simulink model "Demo1"  (R2015a)
settings: Solver=ode45  StartTime=0.0  StopTime=10.0  RelTol=1e-3
InitFcn:
  | Initilization_simulink
values from neighbouring files (symbols this model uses):
  ref = [4.07104996922  -4.5013493727  0; -4.9106735029  -4.17473684081  0; 5.68808751891  0.810273345356  0]    [Config.mat]
undefined symbols (not defined in the file or in its folder): IsPositionTracked, IsSkeletonTracked, JointDepthIndices, JointImageIndices, JointTrackingState, JointWorldCoordinates, none, PositionDepthIndices, PositionImageIndices, PositionWorldCoordinates, SegmentationData, SkeletonTrackingID, videoinput
libraries: imaqlib x1, visionsinks x1
settings Model: CovSFcnEnable=off  Creator=tzwijger  LastModifiedBy=tzwijger
settings DebuggingCC: SolverPrmCheckMsg=warning

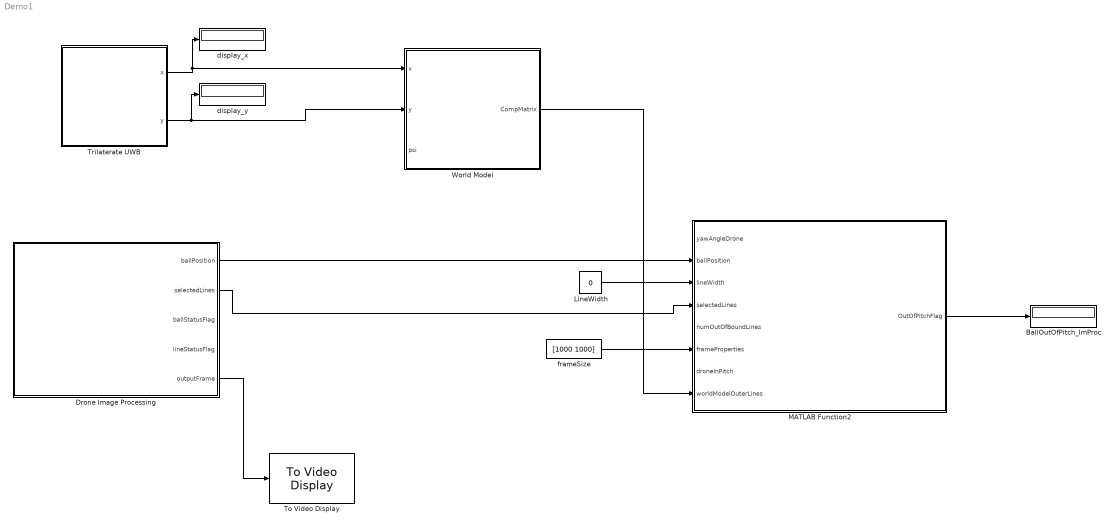
== system Demo1 ==
  BallOutOfPitch_ImProc : Display
  Drone Image Processing : Subsystem
  LineWidth : Constant  Value=0
  MATLAB Function2 : MATLAB Function  TreatAsAtomicUnit=on
  To Video Display : visionsinks/To Video Display  windowSizeMode=True size (1:1)  openAtMdlStart=on  fullScreen=off  videoWindowX=40  videoWindowY=53  saveWindowSize=off  videoWindowWidth=132  videoWindowHeight=41  inputColorFormat=RGB  inputType=Obsolete  imagePorts=One multidimensional signal  OutputDevice=On-screen video monitor  dataOrg=Column-major  isWindowOpen=off
  Trilaterate UWB : Subsystem
  World Model : Subsystem
  display_x : Display
  display_y : Display
  frameSize : Constant  Value=[1000 1000]
  wires:
  Trilaterate UWB/1(x) -> display_x/1, World Model/1(x)
  Trilaterate UWB/2(y) -> World Model/2(y), display_y/1
  Drone Image Processing/5(outputFrame) -> To Video Display/1
  Drone Image Processing/1("ballPosition ") -> MATLAB Function2/2(ballPosition)
  ? -> World Model/3(psi), MATLAB Function2/1(yawAngleDrone)
  LineWidth/1 -> MATLAB Function2/3(lineWidth)
  frameSize/1 -> MATLAB Function2/6(frameProperties)
  ? -> MATLAB Function2/7(droneInPitch)
  MATLAB Function2/1(OutOfPitchFlag) -> BallOutOfPitch_ImProc/1
  Drone Image Processing/2(selectedLines) -> MATLAB Function2/4(selectedLines)
  World Model/1(CompMatrix) -> MATLAB Function2/8(worldModelOuterLines)

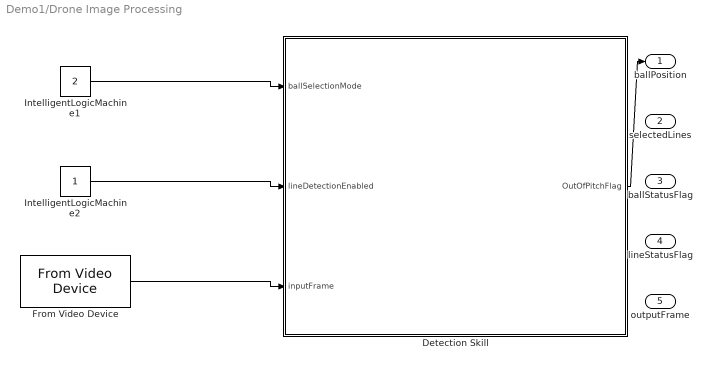
== system Demo1/Drone Image Processing ==
  Detection Skill : MATLAB Function  TreatAsAtomicUnit=on
  From Video Device : imaqlib/From Video Device  DeviceMenu=(none)  Device=winvideo 1 (HP HD Webcam)  ObjConstructor=videoinput('winvideo', 1)  VideoFormatMenu=(none)  VideoFormat=RGB24_640x480  VideoSource=input1  ROIPosition=[0 0 480 640]  EnableHWTrigger=off  TriggerConfiguration=none/none  SampleTime=1/30  OutputPortsMode=One multidimensional signal  DataType=single  CanDoHWTrigger=no  ReturnedColorSpace=rgb  BlockHandle=1921.0006  ROIWidth=640  ROIHeight=480  ROIColumn=0  ROIRow=0  EngXMLPath=C:\Program Files\MATLAB\R2015a\toolbox\imaq\imaq\private  DevXMLPath=C:\Program Files\MATLAB\R2015a\toolbox\imaq\imaqadaptors\win64  EngLibPath=C:\Program Files\MATLAB\R2015a\toolbox\imaq\imaqblks\imaqmex\win64  ColorSpace=rgb  BayerSensorAlignment=grbg  AllMetadata=IsPositionTracked;IsSkeletonTracked;JointDepthIndices;JointImageIndices;JointTrackingState;JointWorldCoordinates;PositionDepthIndices;PositionImageIndices;PositionWorldCoordinates;SegmentationData;SkeletonTrackingID
  IntelligentLogicMachine1 : Constant  Value=2
  IntelligentLogicMachine2 : Constant
  "ballPosition " : Outport
  selectedLines : Outport  Port=2
  ballStatusFlag : Outport  Port=3
  lineStatusFlag : Outport  Port=4
  outputFrame : Outport  Port=5
  wires:
  Detection Skill/1(OutOfPitchFlag) -> "ballPosition "/1
  ? -> outputFrame/1
  ? -> ballStatusFlag/1
  ? -> lineStatusFlag/1
  ? -> selectedLines/1
  IntelligentLogicMachine1/1 -> Detection Skill/1(ballSelectionMode)
  From Video Device/1 -> Detection Skill/3(inputFrame)
  IntelligentLogicMachine2/1 -> Detection Skill/2(lineDetectionEnabled)

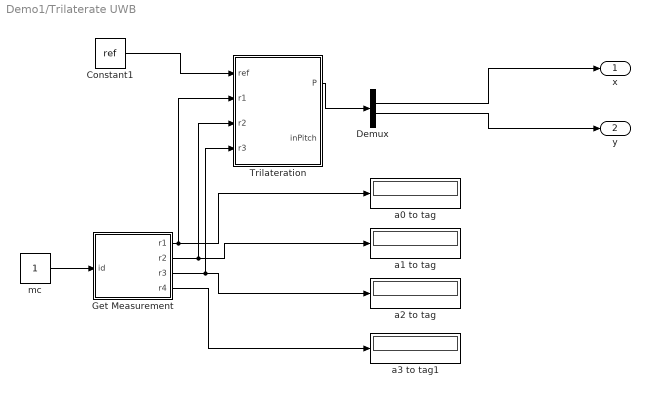
== system Demo1/Trilaterate UWB ==
  Constant1 : Constant  Value=ref
  Demux : Demux
  Get Measurement : MATLAB Function  TreatAsAtomicUnit=on
  Trilateration : MATLAB Function  TreatAsAtomicUnit=on
  a0 to tag : Display
  a1 to tag : Display
  a2 to tag : Display
  a3 to tag1 : Display
  mc : Constant
  x : Outport
  y : Outport  Port=2
  wires:
  Demux/3 -> y/1
  Demux/2 -> x/1
  Trilateration/1(P) -> Demux/1
  Constant1/1 -> Trilateration/1(ref)
  Get Measurement/3(r3) -> a2 to tag/1, Trilateration/4(r3)
  Get Measurement/2(r2) -> a1 to tag/1, Trilateration/3(r2)
  mc/1 -> Get Measurement/1(id)
  Get Measurement/1(r1) -> Trilateration/2(r1), a0 to tag/1
  Get Measurement/4(r4) -> a3 to tag1/1

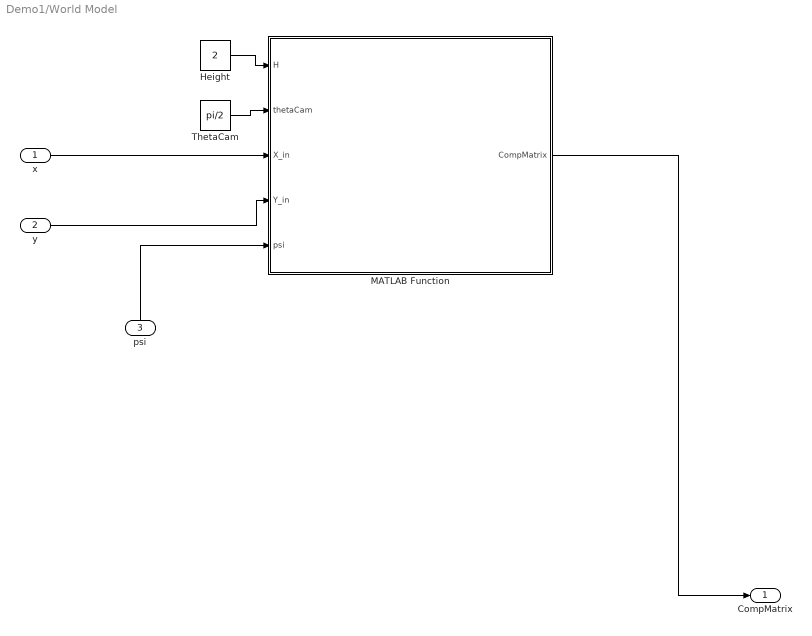
== system Demo1/World Model ==
  x : Inport
  y : Inport  Port=2
  psi : Inport  Port=3
  Height : Constant  Value=2
  MATLAB Function : MATLAB Function  TreatAsAtomicUnit=on
  ThetaCam : Constant  Value=pi/2
  CompMatrix : Outport
  wires:
  MATLAB Function/1(CompMatrix) -> CompMatrix/1
  ThetaCam/1 -> MATLAB Function/2(thetaCam)
  x/1 -> MATLAB Function/3(X_in)
  y/1 -> MATLAB Function/4(Y_in)
  psi/1 -> MATLAB Function/5(psi)
  Height/1 -> MATLAB Function/1(H)

== matlab function Demo1/Trilaterate UWB/Trilateration ==
  data: P output; ref input; r1 input; r2 input; r3 input; inPitch output
function [P, inPitch] = trilateration(ref,r1,r2,r3)%,fign,field2im_params)
% persistent plots k nrplots

coder.extrinsic('Trilateration')

% if isempty(plots)
%     plots = [0];
%     k = 1;
%     nrplots = 10;
% end

P = zeros(4,1);
P = Trilateration(ref',[r1 r2 r3],eye(3));

% % Plot and print results
% [plots, k] = update_plot_trilat(plots, k, fign, P(2:3), field2im_params, nrplots);

== matlab function Demo1/Trilaterate UWB/Get Measurement ==
  data: id input; r1 output; r2 output; r3 output; r4 output
function [r1,r2,r3,r4] = GetMC_sm(id) 
    % Input: Serial Port to A0
    %        
    % Output: Raw data for triangulation
    %
    % Message syntax is explained in the Decawave documentation
    % DecaRangeRTLS_PC_Source_Code_Guide.pdf  - Section 2.3.2
    % DecaRangeRTLS_ARM_Source_Code_Guide.pdf - Section 2.6

    % Make sure to get a measurement with the correct identifier
    persistent s;
    %coder.extrinsic('instrfind','delete','serial','fscanf','strsplit')
    coder.extrinsic('instrfind','delete','serial','fscanf','GetMC')
    
    r1 = 0; r2 = 0; r3 = 0; r4 = 0;
    
    if isempty(s)
        ports = instrfind;
        if ~isempty(ports)
            fclose(ports);
            delete(ports);
        end
        % Establish new connection
        s = serial('COM33','BaudRate',9600,'Parity','None');

        % Open connection
        fopen(s);
        fscanf(s); % Get init mc out of the way and test connection
    end
    
    ids = ['mc';'mr';'ma'];
    id = ids(id,:);
    
    dist = zeros(1,4);
    dist = GetMC(s,id);
    r1 = dist(1);
    r2 = dist(2);
    r3 = dist(3);
    r4 = dist(4); 
end

== matlab function Demo1/World Model/MATLAB Function ==
  data: H input; CompMatrix output; thetaCam input; X_in input; Y_in input; psi input
function CompMatrix   = World(H,thetaCam,X_in,Y_in,psi)

% %field line numbering:  222222222222222222223
%                         1                   3
%                         1                   3
%                         1                   3
%                         1                   3
%                         1                   3
%                         144444444444444444443

% Psi: conter-clock wise positive. zero at localization Y axis
% Theta and rho are defined according to matlab hough transform matrix

Vision=H*tan(thetaCam/2);
X_Vision=Vision;  %<--------------->
Y_Vision=Vision;  %|
                  %|

X=X_in-X_Vision/2;  %moving the origin from center of the camera to top left
Y=-Y_in+Y_Vision/2;
%%%%%%%%%%%%%%%%%%%%%%%%%%%%%%%%%%%%%%%%%%%%%%%%%%%%%%%%%%%%%%%%%%%%%%%%%%
Field_length=8;   %dimentions of the field%<--------------->

Field_width=6; %|
               %|

%%%%%%%%%%%%%%%%%%%%%%%%%%%%%%%%%%%%%%%%%%%%%%%%%%%%%%%%%%%%%%%%%%%%%%%%%%
theta1=(pi)+psi;       %calculate the theta of each side line
theta2=(-pi/2)-psi;
theta3=(0)+psi;
theta4=(pi/2)+psi;
%%%%%%%%%%%%%%%%%%%%%%%%%%%%%%%%%%%%%%%%%%%%%%%%%%%%%%%%%%%%%%%%%%%%%%%%%%%
rho1=abs(X+(Field_length)/2); %calculate rho of each side line with respect to top left cordinate
rho2=abs(Y+(Field_width)/2);
rho3= abs(-X+(Field_length)/2);
rho4= abs(-Y+(Field_width)/2);
%%%%%%%%%%%%%%%%%%%%%%%%%%%%%%%%%%%%%%%%%%%%%%%%%%%%%%%%%%%%%%%%%%%%%%%%
X1=X_in;  %having center to compare the distance and rho
Y1=-Y_in;

rho11=abs(X1+(Field_length)/2);
rho21=abs(Y1+(Field_width)/2);
rho31= abs(-X1+(Field_length)/2);
rho41= abs(-Y1+(Field_width)/2);
%%%%%%%%%%%%%%%%%%%%%%%%%%%%%%%%%%%%%%%%%%%%%%%%%%%%%%%%%%%%%%%%%%%%%%%%%%

Lines=[rho1,theta1,rho11;
rho2,theta2,rho21;
rho3,theta3,rho31;
rho4,theta4,rho41];
B=zeros(4,5);

for k=1:4
    
    i=0;
    rho=Lines(k,1);
    theta=Lines(k,2);
    %if -Y_Vision*sin(theta)<rho &&  rho<X_Vision*cos(theta)
    if Lines(k,3)<X_Vision
        i=1;
        

    end
    if theta>=(2*pi) 
        theta=theta-2*pi;
    end
    if theta<0
        theta=theta+2*pi;
    end
    B(k,:)=[k i 0 rho theta];
end
B(1,3)=2;
B(2,3)=1;
B(3,3)=2;
B(4,3)=1;

CompMatrix=B;

== matlab function Demo1/Drone Image Processing/Detection Skill ==
  data: ballSelectionMode input; OutOfPitchFlag output; lineDetectionEnabled input; inputFrame input
% Author: Nestor Hernandez Rodriguez
% Last Update: 9-03-2016
% Technical University of Eindhoven
% Mechatronic Systems Design PDEng trainee

function OutOfPitchFlag  = detectionSkillAndRefereeing(ballSelectionMode,... 
                                                     lineDetectionEnabled,... 
                                                     inputFrame)
    coder.extrinsic('detectionSkill_V2','refereeingOutOfPitch')
    
    [ballPosition,... 
     selectedLines,... 
     ballStatusFlag,... 
     lineStatusFlag,... 
     outputFrame] = detectionSkill(ballSelectionMode,... 
                                   lineDetectionEnabled,... 
                                   inputFrame);
    
    OutOfPitchFlag  = refereeingOutOfPitch(yawAngleDrone,...
                                           ballPosition,...
                                           lineWidth,...
                                           selectedLines,...
                                           numOutOfBoundLines,...
                                           frameProperties,... 
                                           droneInPitch,...
                                           worldModelOuterLines);
end

== matlab function Demo1/MATLAB Function2 ==
  data: yawAngleDrone input; OutOfPitchFlag output; ballPosition input; lineWidth input; selectedLines input; numOutOfBoundLines input; frameProperties input; droneInPitch input; worldModelOuterLines input
% Author: Nestor Hernandez Rodriguez
% Last Update: 9-03-2016
% Technical University of Eindhoven
% Mechatronic Systems Design PDEng trainee

function OutOfPitchFlag  = refereeingOutOfPitch(yawAngleDrone,ballPosition,lineWidth,selectedLines,numOutOfBoundLines,frameProperties,droneInPitch,worldModelOuterLines)

% This function updates the OutOfPitchFlag ('0'- inside the pitch, '1'-
% out of the pitch or '-1' not known)
% 
% Inputs:
% yawAngleDrone - yaw angle with respect to the field. Should be calibrated
%   so that the outer lines have the initial value as stated in default.
% 
%   Default: goal line yaw angle = pi/2 rad
%            side lines yaw angle = 0 rad
% 
% ballMdl - Object that contains position of the center, diameter and
%   relative position to the selected lines with respect to the frame and
%   taking into account the height of the drone.
% 
% lineWidth - Width of the lines with respect to the frame and taking into
%   account the height of the drone
% 
% selectedLines - Matrix containing the selected lines points, theta and
%   rho [x1_vector y1_vector x2_vector y2_vector theta_vector rho_vector]
% 
% numOutOfBoundLines - Integer that contains the number of outer lines that
%   the frame should contain
%
% frameProperties - [height width] Size of the frame used after pre-process
%
% dronInPitch - Flag '1' - Inside; '0' outside
%
% worldModelOuterLines - Matrix 4x5 containing ID, InFrameFlag, SideOrGoal
% line identification, rho and theta for the 4 outer lines.
%
% The position of the drone within the frame it is assumed to be in the
% center of the frame as it is a top view camera with a pitch angle of 
% pi/2 rad.



mReferenceSideLine = tan(yawAngleDrone); % slope of the side lines
mReferenceGoalLine = tan(yawAngleDrone+pi/2); % slope of the goal lines
mSlopeTH =abs(mReferenceSideLine-mReferenceGoalLine)*0.6; % Threshold slope matching
sizeSelectedLines=size(selectedLines);
rhoDistanceTH=100; % rho threshold 

dronePosition=[frameProperties(1)/2 frameProperties(2)/2];

outOfBoundsDetector=zeros(sizeSelectedLines(1),1); % Create mask for outer lines

auxCntSide=0;
auxCntGoal=0;
auxCnt=0;

% Calculate mask based on slope comparison

for i=1:sizeSelectedLines(1)

    mSlope=(selectedLines(i,4)-selectedLines(i,2))/(selectedLines(i,3)-selectedLines(i,1));
    
    if mSlope>0
        if mSlope<mReferenceSideLine+mSlopeTH && mSlope>mReferenceSideLine-mSlopeTH
            auxCntSide=auxCntSide+1;
            outOfBoundsDetector(i)=1; % '1' for a correct side line matching
        elseif mSlope<mReferenceGoalLine+mSlopeTH && mSlope>mReferenceGoalLine-mSlopeTH
                auxCntGoal=auxCntGoal+1;
                outOfBoundsDetector(i)=2; % '2' for a correct goal line matching
        else
            outOfBoundsDetector(i)=0; % '0' for no matching                    
        end
    else if mSlope>mReferenceSideLine-mSlopeTH && mSlope<mReferenceSideLine+mSlopeTH
            auxCntSide=auxCntSide+1;
            outOfBoundsDetector(i)=1; 
        elseif mSlope>mReferenceGoalLine-mSlopeTH && mSlope<mReferenceGoalLine+mSlopeTH
                auxCntGoal=auxCntGoal+1;
                outOfBoundsDetector(i)=2;            
        else
            outOfBoundsDetector(i)=0; % '0' for no matching
        end
    end            

end 

% Filter possible parallel lines selected as outer lines based on rho provided as input

selectedFilteredLines=zeros(2,6); % First row for possible side line and Second row for possible goal line
auxSideLines=selectedLines(outOfBoundsDetector==1,:);
sizeAuxSideLines=size(auxSideLines);
auxGoalLines=selectedLines(outOfBoundsDetector==2,:);
sizeAuxGoalLines=size(auxGoalLines);

if sizeAuxSideLines(1)>0
    for j=1:sizeAuxSideLines(1)
    %     if auxCntSide>1

        auxWMSideLines=worldModelOuterLines(worldModelOuterLines(:,2)==1,:); % Filter by the InFrameFlag equal to '1'
        auxWMSideLines1=auxWMSideLines(auxWMSideLines(:,3)==1,:); % Filter by the SideOrGoal flag equal to '1' - Side

            if auxSideLines(j,6)>auxWMSideLines1(1,5)-rhoDistanceTH && auxSideLines(j,6)<auxWMSideLines1(1,5)+rhoDistanceTH
                selectedFilteredLines(1,:)=auxSideLines(j,:); % Side line stored in the first row
                auxCntSide=1;
            end
    end
else
   auxCntSide=0;
end

if sizeAuxGoalLines(1)>0
    for j=1:sizeAuxGoalLines(1)
    %     if auxCntSide>1

        auxWMGoalLines=worldModelOuterLines(worldModelOuterLines(:,2)==1,:); % Filter by the InFrameFlag equal to '1'
        auxWMGoalLines1=auxWMGoalLines(auxWMGoalLines(:,3)==2,:); % Filter by the SideOrGoal flag equal to '2' - Side

            if auxGoalLines(j,6)>auxWMGoalLines1(1,5)-rhoDistanceTH && auxGoalLines(j,6)<auxWMGoalLines1(1,5)+rhoDistanceTH
                selectedFilteredLines(2,:)=auxGoalLines(j,:); % Goal line stored in the second row
                auxCntGoal=1;
            end   

    end 
else
   auxCntGoal=0;
end

auxCnt=auxCntSide+auxCntGoal;

% Calculate relative position for ball and drone respect to the filtered outer lines

% Calculate Relative Ball Position
syms x_v2;
sizeFilteredLines=size(selectedFilteredLines);
relativeBallPosition=zeros(sizeFilteredLines(1),1);
relativeDronePosition=zeros(sizeFilteredLines(1),1);

for k=1:sizeFilteredLines(1) % The size of the filtered selected lines
    
    a_p=(selectedFilteredLines(k,4)-selectedFilteredLines(k,2))/(selectedFilteredLines(k,3)-selectedFilteredLines(k,1));
    b_p=(-selectedFilteredLines(k,1)*a_p+selectedFilteredLines(k,2));    
    Fline=symfun(a_p*x_v2+b_p,x_v2);

    % Check position with respect to the lines

    if ballPosition(2)>Fline(ballPosition(1))
        relativeBallPosition(k)= 1; % True (x grows -> right; y grows -> down)
    else
        relativeBallPosition(k)= 0; % False      
    end
end

% Calculate Relative Drone Position

for k=1:sizeFilteredLines(1) % The size of the filtered selected lines
    
    a_p=(selectedFilteredLines(k,4)-selectedFilteredLines(k,2))/(selectedFilteredLines(k,3)-selectedFilteredLines(k,1));
    b_p=(-selectedFilteredLines(k,1)*a_p+selectedFilteredLines(k,2));    
    Fline=symfun(a_p*x_v2+b_p,x_v2);

    % Check position with respect to the lines

    if dronePosition(2)>Fline(dronePosition(1))
        relativeDronePosition(k)= 1; % True (x grows -> right; y grows -> down)
    else
        relativeDronePosition(k)= 0; % False      
    end
end

% Update OutOfBounds flag

switch numOutOfBoundLines
    
    case 2 % Two outer lines can be found (1 Side line and 1 Goal line -> Corner)

        if auxCnt==2 % If this does not match then the refereeing is not done                

           if droneInPitch==1

               if relativeDronePosition(1)==relativeBallPosition(1) && relativeDronePosition(2)==relativeBallPosition(2) % Compare to the 2 outer lines

                   OutOfPitchFlag=0; % Not out of pitch

               else

                   OutOfPitchFlag=1; % Out of pitch
               end
           end
           
        else
            OutOfPitchFlag=-1; % Not known
            
        end

 
    case 1 % One outer line can be found
        
        if auxCnt==1
            if auxCntSide==1
               if droneInPitch==1

                   if relativeDronePosition(1)==relativeBallPosition(1) % Compare to the only outer line

                       OutOfPitchFlag=0; % Not out of pitch

                   else

                       OutOfPitchFlag=1; % Out of pitch
                   end
               end
            else
                if droneInPitch==1

                   if relativeDronePosition(2)==relativeBallPosition(2) % Compare to the only outer line

                       OutOfPitchFlag=0; % Not out of pitch

                   else

                       OutOfPitchFlag=1; % Out of pitch
                   end
                end
            end
           
        else
            OutOfPitchFlag=-1; % Not known
            
        end
    
    otherwise
        
        OutOfPitchFlag=-1; % Not known
        
end
